simulink library "lib_current_control_decoupling"  (R2023a)
settings: Solver=VariableStepAuto  StartTime=0.0  StopTime=10.0  RelTol=1e-3
libraries: lib_conversion x10, lib_configurable_parameter x2
settings Model: Creator=cav2ofo  LastModifiedBy=lenovo
settings OptimizationCC: ReuseModelBlockBuffer=off

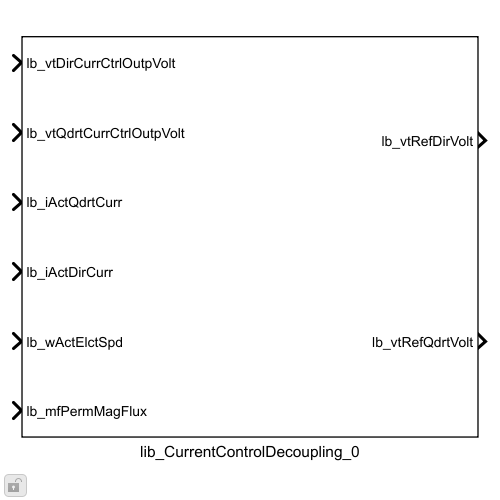
[thumbnail: Simulink's stored preview of the top-level diagram]
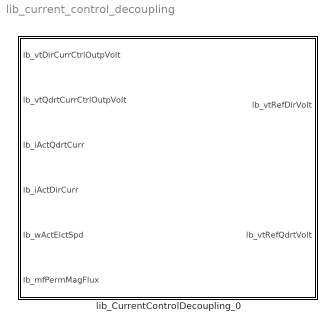
== system lib_current_control_decoupling ==
  lib_CurrentControlDecoupling_0 : Subsystem  mask{lb_parDirIndc=0.0001, lb_parQdrtIndc=0.0001, lb_parMaxPhsIndc=0.001, lb_parMaxElctSpd=4096, lb_parMaxPhsCurr=100, lb_parMaxPermMagFlux=0.01, lb_parMaxCtrlPhsVolt=40, lb_parOutpPekPhy=64, lb_parOutpDataType=fixdt(1,16,2^0,0)}
      mask prompts: lb_parDirIndc "Direct inductance [H]:"; lb_parQdrtIndc "Quadrature inductance [H]:"; lb_parMaxPhsIndc "Maximum phase inductance [H]:"; lb_parMaxElctSpd "Maximum electric speed [rad/s]:"; lb_parMaxPhsCurr "Maximum phase current [A]:"; lb_parMaxPermMagFlux "Maximum permanent magnet flux [Wb]:"; lb_parMaxCtrlPhsVolt "Maximum control phase voltage [V]:"; lb_parOutpPekPhy "Peak output physical value[V]:"; lb_parOutpDataType "Output data type:"
      mask init:
      | %% Define data type for operation w*L
      | lb_parOper1MaxVal = lb_parMaxElctSpd*lb_parMaxPhsIndc;
      | 
      | %% Define data type for operation w*L*I
      | lb_parOper2MaxVal = lb_parMaxElctSpd*lb_parMaxPhsIndc*lb_parMaxPhsCurr;
      | 
      | %% Define data type for operation w*PSI
      | lb_parOper3MaxVal = lb_parMaxElctSpd*lb_parMaxPermMagFlux;
      | 
      | %% Define data type for operation Vc+w*L*I
      | lb_parOper4MaxVal = lb_parMaxCtrlPhsVolt+lb_parMaxElctSpd*lb_parMaxPhsIndc*lb_parMaxPhsCurr;
      | 
      | %% Define data type for operation Vc+w*L*I+w*PSI
      | lb_parOper5MaxVal = lb_parOper4MaxVal+lb_parOper3MaxVal;
      mask DialogControl DescGroupVar Prompt: Current Coupling block
      mask DialogControl DescTextVar Prompt: This block computes the direct and quadrature voltage references.
      mask DialogControl modlPar Prompt: Parameters:
      mask DialogControl modlPar_copy Prompt: Data type:

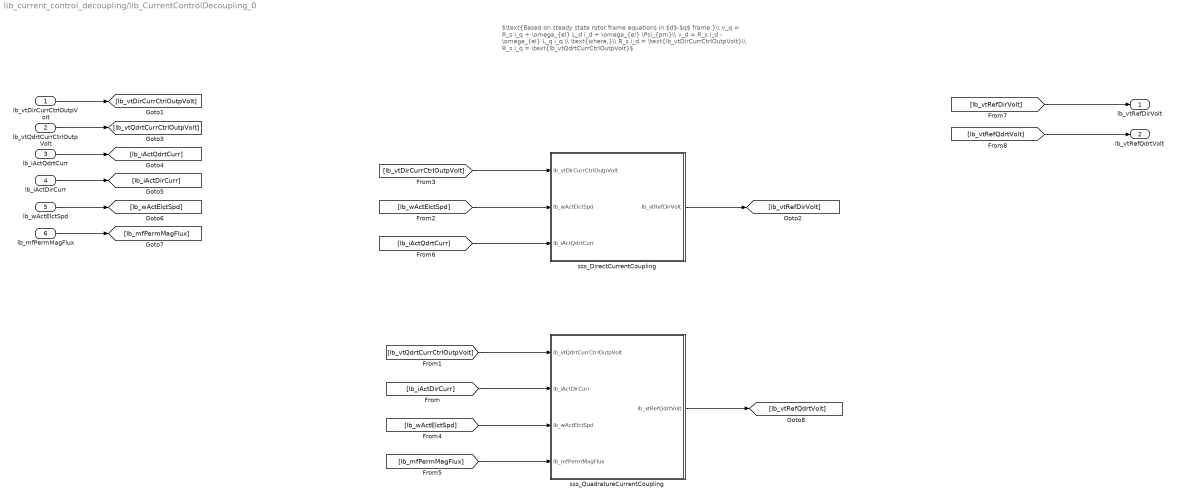
== system lib_current_control_decoupling/lib_CurrentControlDecoupling_0 ==
  note: $\text{Based on steady state rotor frame equations in $d$-$q$ frame:}\\ v_q = R_s i_q + \omega_{el} L_d i_d + \omega_{el} \Psi_{pm}\\ v_d = R_s i_d - \omega_{el} L_q i_q \\ \text{where,}\\ R_s i_d = \text{lb_vtDirCurrCtrlOutpVolt}\\ R_s i_q = \text{lb_vtQdrtCurrCtrlOutpVolt}$
  lb_vtDirCurrCtrlOutpVolt : Inport
  lb_vtQdrtCurrCtrlOutpVolt : Inport  Port=2
  lb_iActQdrtCurr : Inport  Port=3
  lb_iActDirCurr : Inport  Port=4
  lb_wActElctSpd : Inport  Port=5
  lb_mfPermMagFlux : Inport  Port=6
  sss_DirectCurrentCoupling : Subsystem
  sss_QuadratureCurrentCoupling : Subsystem
  lb_vtRefDirVolt : Outport
  lb_vtRefQdrtVolt : Outport  Port=2
  wires:
  [lb_iActDirCurr] -> sss_QuadratureCurrentCoupling/2(lb_iActDirCurr)
  [lb_vtQdrtCurrCtrlOutpVolt] -> sss_QuadratureCurrentCoupling/1(lb_vtQdrtCurrCtrlOutpVolt)
  lb_mfPermMagFlux/1 -> [lb_mfPermMagFlux]
  sss_DirectCurrentCoupling/1(lb_vtRefDirVolt) -> [lb_vtRefDirVolt]
  [lb_vtRefDirVolt] -> lb_vtRefDirVolt/1
  lb_wActElctSpd/1 -> [lb_wActElctSpd]
  [lb_iActQdrtCurr] -> sss_DirectCurrentCoupling/3(lb_iActQdrtCurr)
  [lb_mfPermMagFlux] -> sss_QuadratureCurrentCoupling/4(lb_mfPermMagFlux)
  lb_iActQdrtCurr/1 -> [lb_iActQdrtCurr]
  lb_vtQdrtCurrCtrlOutpVolt/1 -> [lb_vtQdrtCurrCtrlOutpVolt]
  sss_QuadratureCurrentCoupling/1(lb_vtRefQdrtVolt) -> [lb_vtRefQdrtVolt]
  [lb_wActElctSpd] -> sss_DirectCurrentCoupling/2(lb_wActElctSpd)
  [lb_vtRefQdrtVolt] -> lb_vtRefQdrtVolt/1
  lb_iActDirCurr/1 -> [lb_iActDirCurr]
  [lb_vtDirCurrCtrlOutpVolt] -> sss_DirectCurrentCoupling/1(lb_vtDirCurrCtrlOutpVolt)
  lb_vtDirCurrCtrlOutpVolt/1 -> [lb_vtDirCurrCtrlOutpVolt]
  [lb_wActElctSpd] -> sss_QuadratureCurrentCoupling/3(lb_wActElctSpd)

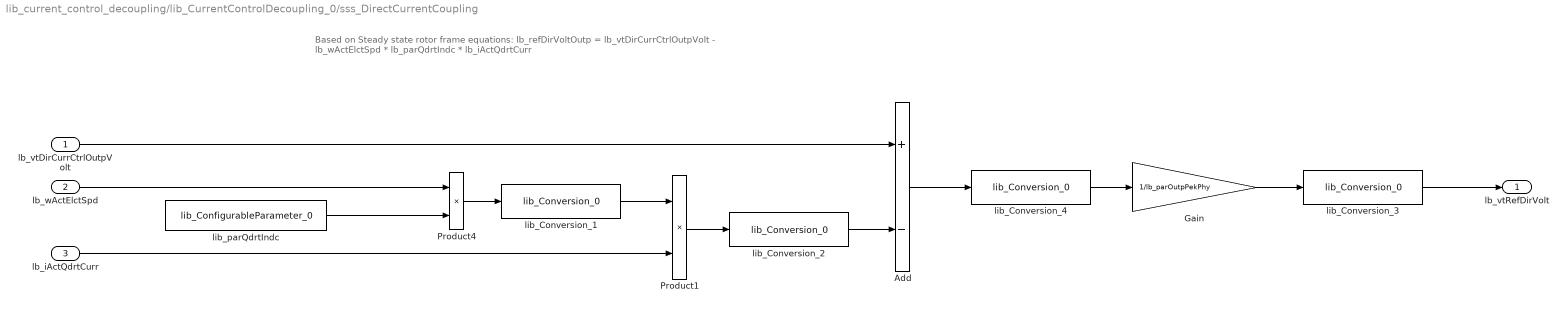
== system lib_current_control_decoupling/lib_CurrentControlDecoupling_0/sss_DirectCurrentCoupling ==
  note: Based on Steady state rotor frame equations:
      |
      | lb_refDirVoltOutp = lb_vtDirCurrCtrlOutpVolt
      | - lb_wActElctSpd * lb_parQdrtIndc * lb_iActQdrtCurr
  lb_vtDirCurrCtrlOutpVolt : Inport
  lb_wActElctSpd : Inport  Port=2
  lb_iActQdrtCurr : Inport  Port=3
  Add : Sum  Inputs=+-  OutDataTypeStr=Inherit: Inherit via back propagation
  Gain : Gain  Gain=1/lb_parOutpPekPhy  OutDataTypeStr=Inherit: Inherit via back propagation
  Product1 : Product  OutDataTypeStr=Inherit: Inherit via back propagation
  Product4 : Product  OutDataTypeStr=Inherit: Inherit via back propagation
  lib_Conversion_1 : lib_conversion/lib_Conversion_0  lb_parDataType=fixdt(1,16)  lb_parOutpMaxVal=lb_parOper1MaxVal  lb_parOutpMinVal=-lb_parOper1MaxVal  lb_parSatFlag=off
  lib_Conversion_2 : lib_conversion/lib_Conversion_0  lb_parDataType=fixdt(1,16)  lb_parOutpMaxVal=lb_parOper2MaxVal  lb_parOutpMinVal=-lb_parOper2MaxVal  lb_parSatFlag=off
  lib_Conversion_3 : lib_conversion/lib_Conversion_0  lb_parDataType=lb_parOutpDataType  lb_parOutpMaxVal=[]  lb_parOutpMinVal=[]  lb_parSatFlag=off
  lib_Conversion_4 : lib_conversion/lib_Conversion_0  lb_parDataType=fixdt(1,16)  lb_parOutpMaxVal=lb_parOper4MaxVal  lb_parOutpMinVal=-lb_parOper4MaxVal  lb_parSatFlag=off
  lib_parQdrtIndc : lib_configurable_parameter/lib_ConfigurableParameter_0  lb_parCnfgPar=lb_parQdrtIndc  lb_parDataType=Inherit: Inherit from 'Constant value'  lb_parUpLim=lb_parMaxPhsIndc  lb_parLowLim=0
  lb_vtRefDirVolt : Outport
  wires:
  lb_wActElctSpd/1 -> Product4/1
  lib_Conversion_2/1 -> Add/2
  lib_Conversion_1/1 -> Product1/1
  Product4/1 -> lib_Conversion_1/1
  lib_Conversion_3/1 -> lb_vtRefDirVolt/1
  Product1/1 -> lib_Conversion_2/1
  lb_iActQdrtCurr/1 -> Product1/2
  lb_vtDirCurrCtrlOutpVolt/1 -> Add/1
  lib_parQdrtIndc/1 -> Product4/2
  lib_Conversion_4/1 -> Gain/1
  Gain/1 -> lib_Conversion_3/1
  Add/1 -> lib_Conversion_4/1

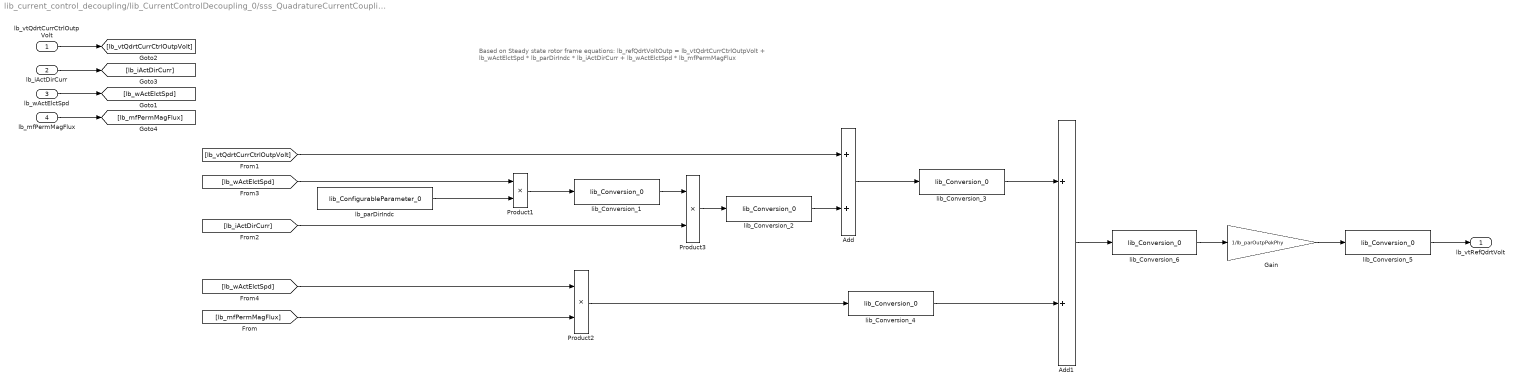
== system lib_current_control_decoupling/lib_CurrentControlDecoupling_0/sss_QuadratureCurrentCoupling ==
  note: Based on Steady state rotor frame equations:
      |
      | lb_refQdrtVoltOutp = lb_vtQdrtCurrCtrlOutpVolt +
      | lb_wActElctSpd * lb_parDirIndc * lb_iActDirCurr +
      | lb_wActElctSpd * lb_mfPermMagFlux
  lb_vtQdrtCurrCtrlOutpVolt : Inport
  lb_iActDirCurr : Inport  Port=2
  lb_wActElctSpd : Inport  Port=3
  lb_mfPermMagFlux : Inport  Port=4
  Add : Sum  OutDataTypeStr=Inherit: Inherit via back propagation
  Add1 : Sum  OutDataTypeStr=Inherit: Inherit via back propagation
  Gain : Gain  Gain=1/lb_parOutpPekPhy  OutDataTypeStr=Inherit: Inherit via back propagation
  Product1 : Product  OutDataTypeStr=Inherit: Inherit via back propagation
  Product2 : Product  OutDataTypeStr=Inherit: Inherit via back propagation
  Product3 : Product  OutDataTypeStr=Inherit: Inherit via back propagation
  lb_parDirIndc : lib_configurable_parameter/lib_ConfigurableParameter_0  lb_parCnfgPar=lb_parDirIndc  lb_parDataType=Inherit: Inherit from 'Constant value'  lb_parUpLim=lb_parMaxPhsIndc  lb_parLowLim=0
  lib_Conversion_1 : lib_conversion/lib_Conversion_0  lb_parDataType=fixdt(1,16)  lb_parOutpMaxVal=lb_parOper1MaxVal  lb_parOutpMinVal=-lb_parOper1MaxVal  lb_parSatFlag=off
  lib_Conversion_2 : lib_conversion/lib_Conversion_0  lb_parDataType=fixdt(1,16)  lb_parOutpMaxVal=lb_parOper2MaxVal  lb_parOutpMinVal=-lb_parOper2MaxVal  lb_parSatFlag=off
  lib_Conversion_3 : lib_conversion/lib_Conversion_0  lb_parDataType=fixdt(1,16)  lb_parOutpMaxVal=lb_parOper4MaxVal  lb_parOutpMinVal=-lb_parOper4MaxVal  lb_parSatFlag=off
  lib_Conversion_4 : lib_conversion/lib_Conversion_0  lb_parDataType=fixdt(1,16)  lb_parOutpMaxVal=lb_parOper3MaxVal  lb_parOutpMinVal=-lb_parOper3MaxVal  lb_parSatFlag=off
  lib_Conversion_5 : lib_conversion/lib_Conversion_0  lb_parDataType=lb_parOutpDataType  lb_parOutpMaxVal=[]  lb_parOutpMinVal=[]  lb_parSatFlag=off
  lib_Conversion_6 : lib_conversion/lib_Conversion_0  lb_parDataType=fixdt(1,16)  lb_parOutpMaxVal=lb_parOper5MaxVal  lb_parOutpMinVal=-lb_parOper5MaxVal  lb_parSatFlag=off
  lb_vtRefQdrtVolt : Outport
  wires:
  lib_Conversion_4/1 -> Add1/2
  Product2/1 -> lib_Conversion_4/1
  lib_Conversion_3/1 -> Add1/1
  Add/1 -> lib_Conversion_3/1
  lib_Conversion_2/1 -> Add/2
  Product3/1 -> lib_Conversion_2/1
  lib_Conversion_1/1 -> Product3/1
  [lb_wActElctSpd] -> Product1/1
  [lb_iActDirCurr] -> Product3/2
  Product1/1 -> lib_Conversion_1/1
  lb_parDirIndc/1 -> Product1/2
  [lb_vtQdrtCurrCtrlOutpVolt] -> Add/1
  [lb_wActElctSpd] -> Product2/1
  [lb_mfPermMagFlux] -> Product2/2
  lib_Conversion_5/1 -> lb_vtRefQdrtVolt/1
  lb_mfPermMagFlux/1 -> [lb_mfPermMagFlux]
  lb_wActElctSpd/1 -> [lb_wActElctSpd]
  lb_iActDirCurr/1 -> [lb_iActDirCurr]
  lb_vtQdrtCurrCtrlOutpVolt/1 -> [lb_vtQdrtCurrCtrlOutpVolt]
  lib_Conversion_6/1 -> Gain/1
  Add1/1 -> lib_Conversion_6/1
  Gain/1 -> lib_Conversion_5/1
